simulink model "servomotor"  (R2024a)
settings: Solver=FixedStepAuto  StartTime=0.0  StopTime=simulationTime  FixedStep=1e-4  RelTol=1e-3
undefined symbols (not defined in the file or in its folder): controller, reference, servo
settings Model: Creator=mmaximo  LastModifiedBy=guilherme
settings SolverCC: AlgebraicLoopSolver=TrustRegion
settings DebuggingCC: UnconnectedInputMsg=warning  UnconnectedOutputMsg=warning  UnconnectedLineMsg=warning
settings ModelReferenceCC: EnableRefExpFcnMdlSchedulingChecks=on
settings RTWCC: GPUComputeCapability=3.5  DLArmComputeVersion=19.05

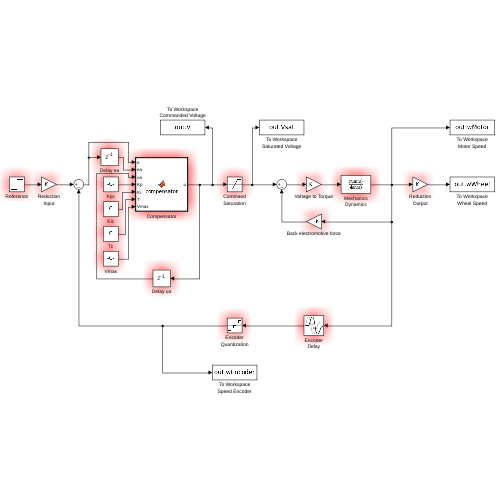
[thumbnail: Simulink's stored preview of the top-level diagram]
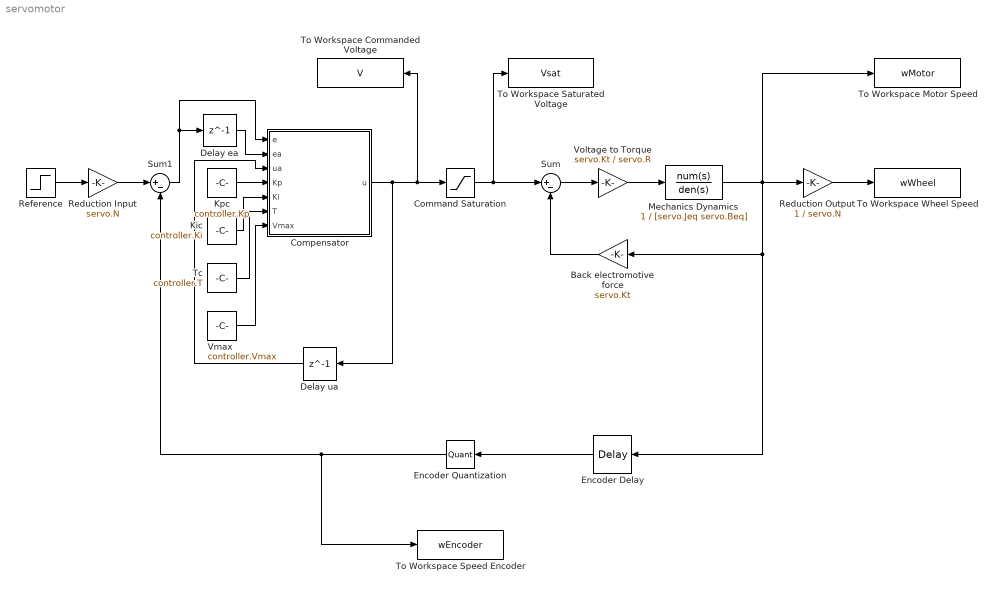
== system servomotor ==
  Back electromotive force : Gain  Gain=servo.Kt
  Command Saturation : Saturate  UpperLimit=servo.Vmax  LowerLimit=-servo.Vmax
  Compensator : MATLAB Function  TreatAsAtomicUnit=on  SystemSampleTime=controller.T
  Delay ea : Delay  DelayLength=1  InitialCondition=0  SampleTime=controller.T
  Delay ua : Delay  DelayLength=1  InitialCondition=0  SampleTime=controller.T
  Encoder Delay : TransportDelay  DelayTime=controller.T / 2.0
  Encoder Quantization : Quantizer  QuantizationInterval=servo.encoderQuantization / controller.T
  Kic : Constant  Value=controller.Ki
  Kpc : Constant  Value=controller.Kp
  Mechanics Dynamics : TransferFcn  Numerator=1  Denominator=[servo.Jeq servo.Beq]
  Reduction Input : Gain  Gain=servo.N
  Reduction Output : Gain  Gain=1 / servo.N
  Reference : Step  Time=reference.stepTime  After=reference.amplitude  SampleTime=0
  Sum : Sum  Inputs=|+-
  Sum1 : Sum  Inputs=|+-
  Tc : Constant  Value=controller.T
  To Workspace Commanded Voltage : ToWorkspace  VariableName=V  SaveFormat=Structure With Time  SampleTime=1e-4
  To Workspace Motor Speed : ToWorkspace  VariableName=wMotor  SaveFormat=Structure With Time  SampleTime=1e-4
  To Workspace Saturated Voltage : ToWorkspace  VariableName=Vsat  SaveFormat=Structure With Time  SampleTime=1e-4
  To Workspace Speed Encoder : ToWorkspace  VariableName=wEncoder  SaveFormat=Structure With Time  SampleTime=1e-4
  To Workspace Wheel Speed : ToWorkspace  VariableName=wWheel  SaveFormat=Structure With Time  SampleTime=1e-4
  Vmax : Constant  Value=controller.Vmax
  Voltage to Torque : Gain  Gain=servo.Kt / servo.R
  wires:
  Back electromotive force/1 -> Sum/2
  Sum/1 -> Voltage to Torque/1
  Mechanics Dynamics/1 -> Reduction Output/1, To Workspace Motor Speed/1, Encoder Delay/1, Back electromotive force/1
  Reference/1 -> Reduction Input/1
  Reduction Output/1 -> To Workspace Wheel Speed/1
  Voltage to Torque/1 -> Mechanics Dynamics/1
  Compensator/1(u) -> Delay ua/1, To Workspace Commanded Voltage/1, Command Saturation/1
  Command Saturation/1 -> Sum/1, To Workspace Saturated Voltage/1
  Reduction Input/1 -> Sum1/1
  Encoder Delay/1 -> Encoder Quantization/1
  Encoder Quantization/1 -> Sum1/2, To Workspace Speed Encoder/1
  Kic/1 -> Compensator/5(Ki)
  Vmax/1 -> Compensator/7(Vmax)
  Tc/1 -> Compensator/6(T)
  Kpc/1 -> Compensator/4(Kp)
  Sum1/1 -> Compensator/1(e), Delay ea/1
  Delay ua/1 -> Compensator/3(ua)
  Delay ea/1 -> Compensator/2(ea)

== matlab function servomotor/Compensator ==
  data: e input; u output; ea input; ua input; Kp input; Ki input; T input; Vmax input
function u = compensator(e, ea, ua, Kp, Ki, T, Vmax)
% u = compensator(e, ea, ua, Kp, Ki, T, Vmax)
% Implements the PI discrete compensator.
% Inputs:
% e: current error e[k].
% ea: previous error e[k-1].
% ua: previous command u[k-1].
% Kp: proportional gain.
% Ki: integrative gain.
% T: sample time.
% Vmax: voltage limit.
% Output:
% u: current command u[k].

% Digital control law
u = ua + (Kp + Ki * T / 2) * e + (-Kp + Ki * T / 2) * ea;

% Anti-windup
if u < -Vmax
    u = -Vmax;
elseif u > Vmax
    u = Vmax;
end

end
